simulink model "UR_BS_only_pos"  (R2022a)
settings: Solver=VariableStepAuto  StartTime=0.0  StopTime=200  RelTol=1e-6
undefined symbols (not defined in the file): DiscIntNeverNeededParam, dq0, Ks_BS, Levenberg, Marquardt, p0, q0, r0, r1, r2, rel_err, slow
libraries: robotmaniplib x4, simulink x1
settings Model: PauseTimes=0.14  Creator=Mathew  LastModifiedBy=Marco
settings SolverCC: ZeroCrossControl=DisableAll  ODENIntegrationMethod=ode1be
settings DebuggingCC: AlgebraicLoopMsg=none  UnconnectedInputMsg=warning  UnconnectedOutputMsg=warning  UnconnectedLineMsg=warning  SFMachineParentedDataDiag=warning
settings SFSimCC: CustomCodeUndefinedFunction=UseInterfaceOnly
settings RTWCC: DLArmComputeVersion=19.05

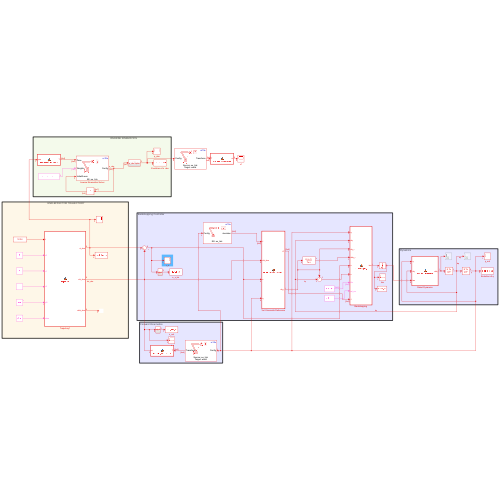
[thumbnail: Simulink's stored preview of the top-level diagram]
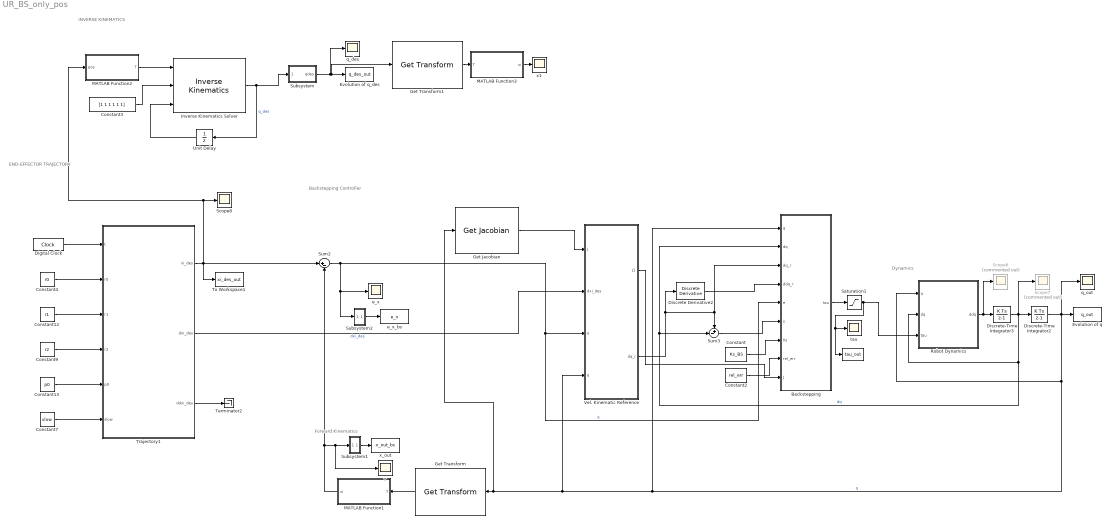
== system UR_BS_only_pos ==
  note: Backstepping Controller
  note: Forward Kinematics
  note: Dynamics
  note: INVERSE KINEMATICS
  note: END-EFFECTOR TRAJECTORY
  "         " : ToWorkspace  VariableName=tau_out  SaveFormat=Timeseries  SampleTime=-1
  Backstepping : MATLAB Function  TreatAsAtomicUnit=on
  Constant : Constant  Value=Ks_BS
  Constant12 : Constant  Value=r1
  Constant13 : Constant  Value=p0
  Constant2 : Constant  Value=rel_err
  Constant3 : Constant  Value=[1 1 1 1 1 1]
  Constant4 : Constant  Value=r0
  Constant7 : Constant  Value=slow
  Constant9 : Constant  Value=r2
  Digital Clock : DigitalClock  SampleTime=0.01
  Discrete Derivative2 : simulink/Discrete/Discrete Derivative  gainval=1.0  ICPrevScaledInput=ddq0  OutMin=[]  OutMax=[]  OutDataType=fixdt(1, 16)  OutScaling=2^-10  DoSatur=off
  Discrete-Time Integrator2 : DiscreteIntegrator  InitialCondition=q0  SampleTime=-1  ICPrevOutput=DiscIntNeverNeededParam  ICPrevScaledInput=DiscIntNeverNeededParam
  Discrete-Time Integrator3 : DiscreteIntegrator  InitialCondition=dq0  SampleTime=-1  ICPrevOutput=DiscIntNeverNeededParam  ICPrevScaledInput=DiscIntNeverNeededParam
  Evolution of q : ToWorkspace  VariableName=q_out  SaveFormat=Timeseries  SampleTime=-1
  Evolution of q_des : ToWorkspace  VariableName=q_des_out  SaveFormat=Timeseries  SampleTime=-1
  Get Jacobian : robotmaniplib/Get Jacobian  RigidBodyTree=ur10e  EndEffector=ee_link  SimulateUsing=Interpreted execution
      settings: SourceProductBaseCode=RO
  Get Transform : robotmaniplib/Get Transform  RigidBodyTree=ur10e  SourceBody=ee_link  TargetBody=world  SimulateUsing=Interpreted execution
  Get Transform1 : robotmaniplib/Get Transform  RigidBodyTree=ur10e  SourceBody=ee_link  TargetBody=world  SimulateUsing=Interpreted execution
  Inverse Kinematics Solver : robotmaniplib/Inverse Kinematics  RigidBodyTree=ur10e  EndEffector=ee_link  ShowInfo=off  SolverName=Levenberg-Marquardt  EnforceJointLimits=on  MaxIterations=1500  MaxTime=10  GradientTolerance=1e-7  SolutionTolerance=1e-5  StepTolerance=1e-14  ErrorChangeTolerance=1e-8  UseErrorDamping=on  DampingBias=0.0025  SimulateUsing=Interpreted execution
  MATLAB Function1 : MATLAB Function  TreatAsAtomicUnit=on
  MATLAB Function2 : MATLAB Function  TreatAsAtomicUnit=on
  MATLAB Function3 : MATLAB Function  TreatAsAtomicUnit=on
  Robot Dynamics : MATLAB Function  TreatAsAtomicUnit=on
  Saturation1 : Saturate  UpperLimit=100  LowerLimit=-100
  Scope6 : Scope  Commented=on
  Scope7 : Scope  Commented=on
  Scope8 : Scope
  Subsystem : Subsystem
  Subsystem1 : Subsystem
  Subsystem2 : Subsystem
  Sum2 : Sum  Inputs=|+-
  Sum3 : Sum  Inputs=+-|
  Terminator2 : Terminator
  To Workspace1 : ToWorkspace  VariableName=xi_des_out  SaveFormat=Timeseries  SampleTime=-1
  Trajectory1 : MATLAB Function  TreatAsAtomicUnit=on
  Unit Delay : UnitDelay  SampleTime=-1  HasFrameUpgradeWarning=on
  "Vel. Kinematic Reference " : MATLAB Function  TreatAsAtomicUnit=on
  e_x : Scope
  e_x_bs : ToWorkspace  VariableName=e_x  SaveFormat=Timeseries  SampleTime=-1
  q_des : Scope
  q_out : Scope
  tau : Scope
  x : Scope
  x1 : Scope
  x_out : ToWorkspace  VariableName=x_out_bs  SaveFormat=Timeseries  SampleTime=-1
  wires:
  Discrete-Time Integrator3/1 -> Scope7/1, Discrete-Time Integrator2/1, Backstepping/2(dq), Sum3/2, Robot Dynamics/2(dq)  "dq"
  Discrete-Time Integrator2/1 -> q_out/1, Evolution of q/1, Backstepping/1(q), "Vel. Kinematic Reference "/4(q), Get Jacobian/1, Get Transform/1, Robot Dynamics/1(q)  "q"
  Robot Dynamics/1(ddq) -> Scope6/1, Discrete-Time Integrator3/1
  Constant/1 -> Backstepping/7(Ks)
  Constant2/1 -> Backstepping/8(rel_err)
  Backstepping/1(tau) -> Saturation1/1
  Saturation1/1 -> Robot Dynamics/3(tau), tau/1, "         "/1
  Inverse Kinematics Solver/1 -> Subsystem/1(q_des), Unit Delay/1  "q_des"
  Constant4/1 -> Trajectory1/2(r0)
  Trajectory1/2(dxi_des) -> "Vel. Kinematic Reference "/2(dxi_des)  "dxi_des"
  Digital Clock/1 -> Trajectory1/1(t)
  Unit Delay/1 -> Inverse Kinematics Solver/3
  MATLAB Function2/1(T) -> Inverse Kinematics Solver/1
  Constant3/1 -> Inverse Kinematics Solver/2
  Trajectory1/3(ddxi_des) -> Terminator2/1
  Constant12/1 -> Trajectory1/3(r1)
  Constant9/1 -> Trajectory1/4(r2)
  Constant7/1 -> Trajectory1/6(slow)
  Constant13/1 -> Trajectory1/5(p0)
  Trajectory1/1(xi_des) -> To Workspace1/1, Sum2/1, MATLAB Function2/1(pos), Scope8/1
  "Vel. Kinematic Reference "/2(dq_r) -> Backstepping/3(dq_r), Sum3/1, Discrete Derivative2/1
  Get Jacobian/1 -> "Vel. Kinematic Reference "/1(J)
  Subsystem1/1(qdes) -> x_out/1
  MATLAB Function1/1(xi) -> Sum2/2, Subsystem1/1(q_des), x/1
  Subsystem2/1(qdes) -> e_x_bs/1
  Sum2/1 -> "Vel. Kinematic Reference "/3(e), Backstepping/5(e), Subsystem2/1(q_des), e_x/1  "e"
  Get Transform/1 -> MATLAB Function1/1(T)
  Discrete Derivative2/1 -> Backstepping/4(ddq_r)
  Sum3/1 -> Backstepping/6(s)
  Get Transform1/1 -> MATLAB Function3/1(T)
  Subsystem/1(qdes) -> q_des/1, Get Transform1/1, Evolution of q_des/1
  MATLAB Function3/1(xi) -> x1/1
  "Vel. Kinematic Reference "/1(J1) -> Backstepping/9(J)

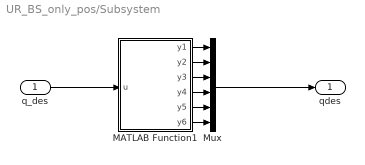
== system UR_BS_only_pos/Subsystem ==
  q_des : Inport
  MATLAB Function1 : MATLAB Function  TreatAsAtomicUnit=on
  Mux : Mux  Inputs=6
  qdes : Outport
  wires:
  MATLAB Function1/5(y5) -> Mux/5
  MATLAB Function1/1(y1) -> Mux/1
  Mux/1 -> qdes/1
  MATLAB Function1/4(y4) -> Mux/4
  MATLAB Function1/6(y6) -> Mux/6
  q_des/1 -> MATLAB Function1/1(u)
  MATLAB Function1/2(y2) -> Mux/2
  MATLAB Function1/3(y3) -> Mux/3

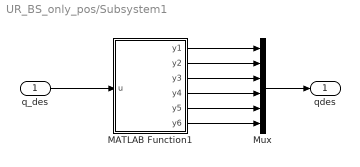
== system UR_BS_only_pos/Subsystem1 ==
  q_des : Inport
  MATLAB Function1 : MATLAB Function  TreatAsAtomicUnit=on
  Mux : Mux  Inputs=6
  qdes : Outport
  wires:
  MATLAB Function1/6(y6) -> Mux/6
  MATLAB Function1/5(y5) -> Mux/5
  MATLAB Function1/4(y4) -> Mux/4
  MATLAB Function1/3(y3) -> Mux/3
  MATLAB Function1/2(y2) -> Mux/2
  q_des/1 -> MATLAB Function1/1(u)
  Mux/1 -> qdes/1
  MATLAB Function1/1(y1) -> Mux/1

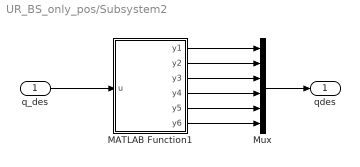
== system UR_BS_only_pos/Subsystem2 ==
  q_des : Inport
  MATLAB Function1 : MATLAB Function  TreatAsAtomicUnit=on
  Mux : Mux  Inputs=6
  qdes : Outport
  wires:
  MATLAB Function1/1(y1) -> Mux/1
  Mux/1 -> qdes/1
  q_des/1 -> MATLAB Function1/1(u)
  MATLAB Function1/2(y2) -> Mux/2
  MATLAB Function1/3(y3) -> Mux/3
  MATLAB Function1/4(y4) -> Mux/4
  MATLAB Function1/5(y5) -> Mux/5
  MATLAB Function1/6(y6) -> Mux/6

== matlab function UR_BS_only_pos/MATLAB Function2 ==
  data: pos input; T output
function T = homogeneus_transf(pos)

R=eye(3);
T=eye(4);

% Use a XYZ parametrization for pose determination

% R = eul2rotm([pos(4);pos(5);pos(6)], 'XYZ');

phi   = pos(4);
theta = pos(5);
psi   = pos(6);

R = [                              cos(psi)*cos(theta),                             -cos(theta)*sin(psi),           sin(theta) ;
     cos(phi)*sin(psi) + cos(psi)*sin(phi)*sin(theta), cos(phi)*cos(psi) - sin(phi)*sin(psi)*sin(theta), -cos(theta)*sin(phi)  ;
     sin(phi)*sin(psi) - cos(phi)*cos(psi)*sin(theta), cos(psi)*sin(phi) + cos(phi)*sin(psi)*sin(theta),  cos(phi)*cos(theta)] ;

T = [  R,     [pos(1);pos(2);pos(3) ];
     0 0 0              1           ]; 

end

== matlab function UR_BS_only_pos/Robot Dynamics ==
  data: q input; dq input; tau input; ddq output
function ddq = inverse_dynamics(q, dq, tau)
    
    g = 9.81;
    
    % Get dynamic matrices
    M = UR_B(q);
    C = UR_C(q, dq);
    G = UR_G(q,g);
    
    ddq = pinv(M)*(tau - C*dq - G);

end

== matlab function UR_BS_only_pos/MATLAB Function3 ==
  data: T input; xi output
function xi   = forward_kinematics(T)

%   [T,phi,theta,psi] = UR_FK(q);
    
    R = T(1:3,1:3);
    eulXYZ = rotm2eul(R, 'XYZ');
    phi   = eulXYZ(1);
    theta = eulXYZ(2);
    psi   = eulXYZ(3);
    
    xi = [T(1:3,4);phi;theta;psi];

end

== matlab function UR_BS_only_pos/MATLAB Function1 ==
  data: T input; xi output
function xi   = forward_kinematics(T)

%   [T,phi,theta,psi] = UR_FK(q);
    
    R = T(1:3,1:3);
    eulXYZ = rotm2eul(R, 'XYZ');
    phi   = eulXYZ(1);
    theta = eulXYZ(2);
    psi   = eulXYZ(3);
    
    xi = [T(1:3,4);phi;theta;psi];

end

== matlab function UR_BS_only_pos/Vel. Kinematic Reference  ==
  data: J1 output; J input; dxi_des input; dq_r output; e input; q input; Lambda_BS parameter
function [J1,dq_r] = vel_kinematic_reference(J, dxi_des, e, q, Lambda_BS)

    % Computing jacobian
    J1 = J(4:6,1:6);
     
    dq_r = pinv(J1) * (dxi_des(1:3) + Lambda_BS(1:3,1:3)*e(1:3));


end

== matlab function UR_BS_only_pos/Subsystem/MATLAB Function1 ==
  data: u input; y1 output; y2 output; y3 output; y4 output; y5 output; y6 output
function [y1,y2,y3,y4,y5,y6] = fcn(u)

y1 = squeeze(u(1));
y2 = squeeze(u(2));
y3 = squeeze(u(3));
y4 = squeeze(u(4));
y5 = squeeze(u(5));
y6 = squeeze(u(6));

== matlab function UR_BS_only_pos/Backstepping ==
  data: q input; dq input; dq_r input; tau output; ddq_r input; e input; s input; Ks input; rel_err input; J input
function tau = backstepping(q, dq, dq_r, ddq_r, e, s, Ks, rel_err,J)

    g = 9.81;
    
%      J = J(4:6,1:3);
%     J=[J1(4:6,1:6);J1(1:3,1:6)];

    % Get dynamic matrices
    M = UR_B(q);
    C = UR_C(q,dq);
    G = UR_G(q,g);
    
    % Adding uncertainty
    M = M.*(1 + rel_err);
    C = C.*(1 + rel_err);
    G = G.*(1 + rel_err);
    
    % Control law
    tau = M*ddq_r + C*dq_r + G + Ks*s + J.'*e(1:3);

end

== matlab function UR_BS_only_pos/Trajectory1 ==
  data: t input; r0 input; xi_des output; r1 input; r2 input; p0 input; slow input; dxi_des output; ddxi_des output
function [xi_des, dxi_des, ddxi_des] = trajectory(t,r0,r1,r2,p0,slow)

k=slow;

xi_des =   [r0*sin(t/(2*k))       ; r1*sin(t/k)     ; r2*cos(t/k)     ;0;0;0] + p0;
dxi_des =  [r0/2/k*cos(t/(2*k))   ; r1/k*cos(t/k)   ; -r2/k*sin(t/k)  ;0;0;0];
ddxi_des = [-r0/4/k/k*sin(t/(2*k)); -r1/k/k*sin(t/k); -r2/k/k*cos(t/k);0;0;0];

== matlab function UR_BS_only_pos/Subsystem1/MATLAB Function1 ==
  data: u input; y1 output; y2 output; y3 output; y4 output; y5 output; y6 output
function [y1,y2,y3,y4,y5,y6] = fcn(u)

y1 = squeeze(u(1));
y2 = squeeze(u(2));
y3 = squeeze(u(3));
y4 = squeeze(u(4));
y5 = squeeze(u(5));
y6 = squeeze(u(6));

== matlab function UR_BS_only_pos/Subsystem2/MATLAB Function1 ==
  data: u input; y1 output; y2 output; y3 output; y4 output; y5 output; y6 output
function [y1,y2,y3,y4,y5,y6] = fcn(u)

y1 = squeeze(u(1));
y2 = squeeze(u(2));
y3 = squeeze(u(3));
y4 = squeeze(u(4));
y5 = squeeze(u(5));
y6 = squeeze(u(6));
